simulink model "CACC"  (R2018a)
settings: Solver=VariableStepAuto  StartTime=0.0  StopTime=100  RelTol=1e-3
libraries: cstblocks x7
settings Model: Creator=uzeyi  LastModifiedBy=uzeyi

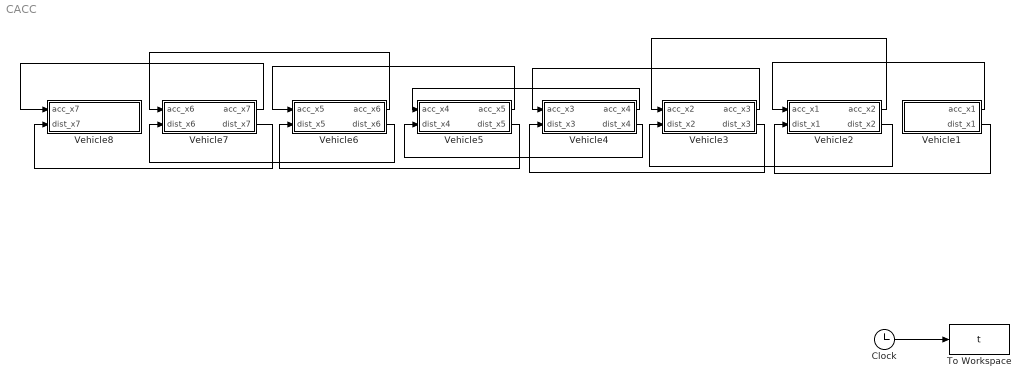
== system CACC ==
  Clock : Clock
  To Workspace : ToWorkspace  VariableName=t  SampleTime=-1
  Vehicle1 : Subsystem
  Vehicle2 : Subsystem
  Vehicle3 : Subsystem
  Vehicle4 : Subsystem
  Vehicle5 : Subsystem
  Vehicle6 : Subsystem
  Vehicle7 : Subsystem
  Vehicle8 : Subsystem
  wires:
  Vehicle1/2(dist_x1) -> Vehicle2/2(dist_x1)
  Clock/1 -> To Workspace/1
  Vehicle2/2(dist_x2) -> Vehicle3/2(dist_x2)
  Vehicle1/1("acc_x1 ") -> Vehicle2/1("acc_x1 ")
  Vehicle2/1(acc_x2) -> Vehicle3/1("acc_x2 ")
  Vehicle3/2(dist_x3) -> Vehicle4/2(dist_x3)
  Vehicle3/1(acc_x3) -> Vehicle4/1("acc_x3 ")
  Vehicle4/2(dist_x4) -> Vehicle5/2(dist_x4)
  Vehicle4/1(acc_x4) -> Vehicle5/1("acc_x4 ")
  Vehicle5/2(dist_x5) -> Vehicle6/2(dist_x5)
  Vehicle5/1(acc_x5) -> Vehicle6/1("acc_x5 ")
  Vehicle6/1(acc_x6) -> Vehicle7/1("acc_x6 ")
  Vehicle7/2(dist_x7) -> Vehicle8/2(dist_x7)
  Vehicle7/1(acc_x7) -> Vehicle8/1("acc_x7 ")
  Vehicle6/2(dist_x6) -> Vehicle7/2(dist_x6)

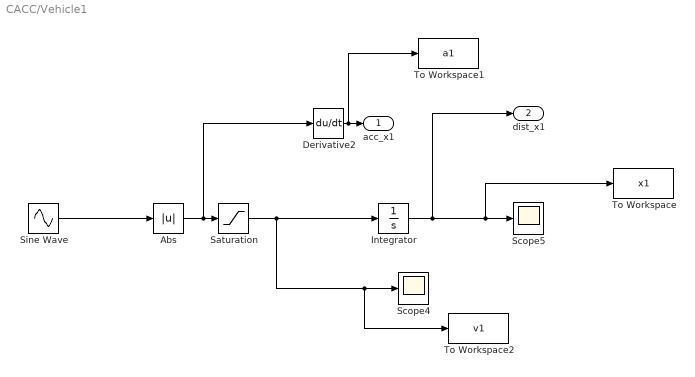
== system CACC/Vehicle1 ==
  Abs : Abs
  Derivative2 : Derivative
  Integrator : Integrator  InitialCondition=80
  Saturation : Saturate  UpperLimit=10  LowerLimit=5
  Scope4 : Scope
  Scope5 : Scope
  Sine Wave : Sin  Amplitude=10  SampleTime=0
  To Workspace : ToWorkspace  VariableName=x1  SampleTime=-1
  To Workspace1 : ToWorkspace  VariableName=a1  SampleTime=-1
  To Workspace2 : ToWorkspace  VariableName=v1  SampleTime=-1
  "acc_x1 " : Outport
  dist_x1 : Outport  Port=2
  wires:
  Sine Wave/1 -> Abs/1
  Saturation/1 -> To Workspace2/1, Scope4/1, Integrator/1
  Integrator/1 -> dist_x1/1, To Workspace/1, Scope5/1
  Derivative2/1 -> To Workspace1/1, "acc_x1 "/1
  Abs/1 -> Derivative2/1, Saturation/1

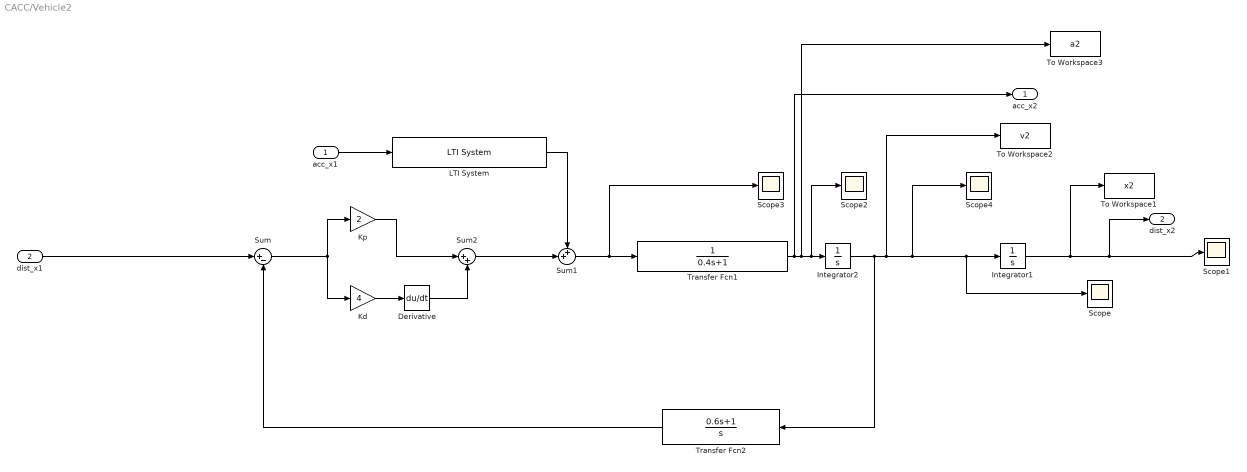
== system CACC/Vehicle2 ==
  "acc_x1 " : Inport
  dist_x1 : Inport  Port=2
  Derivative : Derivative
  Integrator1 : Integrator  InitialCondition=70  IgnoreLimit=on
  Integrator2 : Integrator  InitialCondition=1  IgnoreLimit=on
  Kd : Gain  Gain=4
  Kp : Gain  Gain=2
  LTI System : cstblocks/LTI System  sys=tf([0.4 1],[0.6 1],'InputDelay',0.3)  IC=[]
  Scope{,1..4} (5 alike) : Scope
  Sum : Sum  Inputs=|+-
  Sum1 : Sum  Inputs=++|
  Sum2 : Sum  Inputs=|++
  To Workspace1 : ToWorkspace  VariableName=x2  SampleTime=-1
  To Workspace2 : ToWorkspace  VariableName=v2  SampleTime=-1
  To Workspace3 : ToWorkspace  VariableName=a2  SampleTime=-1
  Transfer Fcn1 : TransferFcn  Denominator=[0.4 1 ]
  Transfer Fcn2 : TransferFcn  Numerator=[0.6 1]  Denominator=[1 0]
  acc_x2 : Outport
  dist_x2 : Outport  Port=2
  wires:
  Kd/1 -> Derivative/1
  LTI System/1 -> Sum1/1
  dist_x1/1 -> Sum/1
  Transfer Fcn1/1 -> acc_x2/1, To Workspace3/1, Scope2/1, Integrator2/1
  Transfer Fcn2/1 -> Sum/2
  Kp/1 -> Sum2/1
  "acc_x1 "/1 -> LTI System/1
  Integrator1/1 -> To Workspace1/1, dist_x2/1, Scope1/1
  Sum/1 -> Kp/1, Kd/1
  Integrator2/1 -> Transfer Fcn2/1, To Workspace2/1, Scope4/1, Scope/1, Integrator1/1
  Derivative/1 -> Sum2/2
  Sum1/1 -> Scope3/1, Transfer Fcn1/1
  Sum2/1 -> Sum1/2

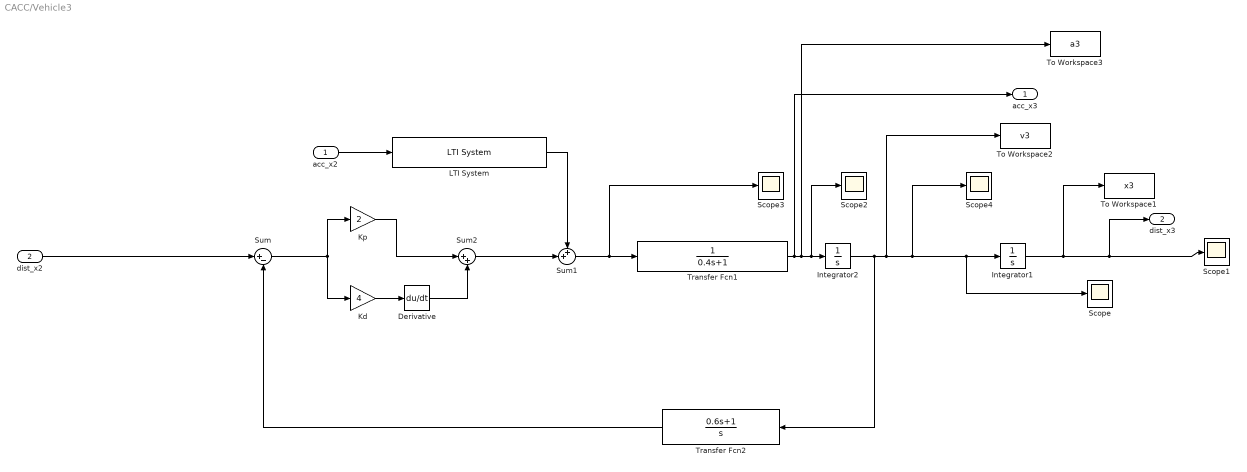
== system CACC/Vehicle3 ==
  "acc_x2 " : Inport
  dist_x2 : Inport  Port=2
  Derivative : Derivative
  Integrator1 : Integrator  InitialCondition=60  IgnoreLimit=on
  Integrator2 : Integrator  InitialCondition=1  IgnoreLimit=on
  Kd : Gain  Gain=4
  Kp : Gain  Gain=2
  LTI System : cstblocks/LTI System  sys=tf([0.4 1],[0.6 1],'InputDelay',0.3)  IC=[]
  Scope{,1..4} (5 alike) : Scope
  Sum : Sum  Inputs=|+-
  Sum1 : Sum  Inputs=++|
  Sum2 : Sum  Inputs=|++
  To Workspace1 : ToWorkspace  VariableName=x3  SampleTime=-1
  To Workspace2 : ToWorkspace  VariableName=v3  SampleTime=-1
  To Workspace3 : ToWorkspace  VariableName=a3  SampleTime=-1
  Transfer Fcn1 : TransferFcn  Denominator=[0.4 1 ]
  Transfer Fcn2 : TransferFcn  Numerator=[0.6 1]  Denominator=[1 0]
  acc_x3 : Outport
  dist_x3 : Outport  Port=2
  wires:
  Kd/1 -> Derivative/1
  LTI System/1 -> Sum1/1
  dist_x2/1 -> Sum/1
  Transfer Fcn1/1 -> acc_x3/1, To Workspace3/1, Scope2/1, Integrator2/1
  Transfer Fcn2/1 -> Sum/2
  Kp/1 -> Sum2/1
  "acc_x2 "/1 -> LTI System/1
  Integrator1/1 -> To Workspace1/1, dist_x3/1, Scope1/1
  Sum/1 -> Kp/1, Kd/1
  Integrator2/1 -> Transfer Fcn2/1, To Workspace2/1, Scope4/1, Scope/1, Integrator1/1
  Derivative/1 -> Sum2/2
  Sum1/1 -> Scope3/1, Transfer Fcn1/1
  Sum2/1 -> Sum1/2

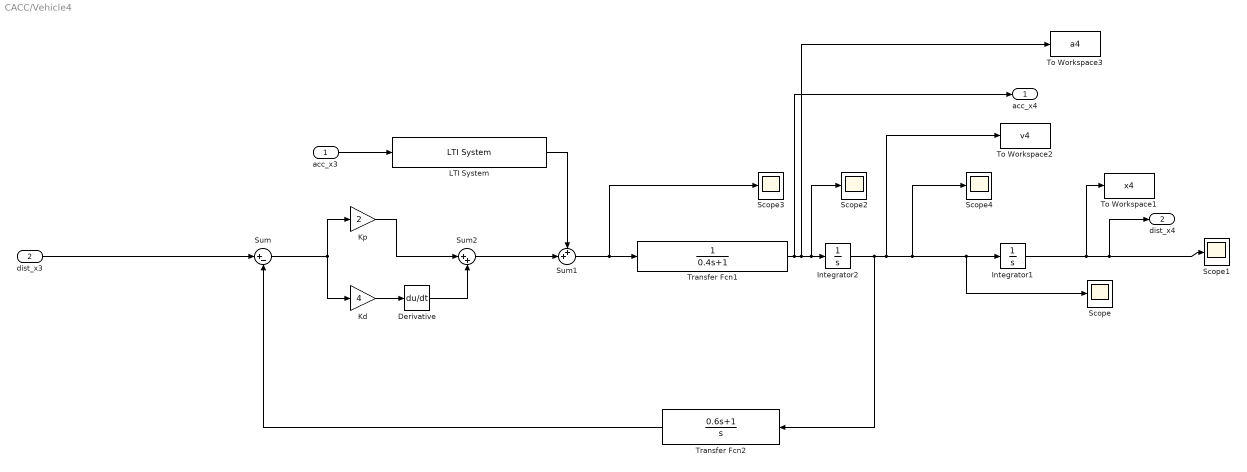
== system CACC/Vehicle4 ==
  "acc_x3 " : Inport
  dist_x3 : Inport  Port=2
  Derivative : Derivative
  Integrator1 : Integrator  InitialCondition=50  IgnoreLimit=on
  Integrator2 : Integrator  InitialCondition=1  IgnoreLimit=on
  Kd : Gain  Gain=4
  Kp : Gain  Gain=2
  LTI System : cstblocks/LTI System  sys=tf([0.4 1],[0.6 1],'InputDelay',0.3)  IC=[]
  Scope{,1..4} (5 alike) : Scope
  Sum : Sum  Inputs=|+-
  Sum1 : Sum  Inputs=++|
  Sum2 : Sum  Inputs=|++
  To Workspace1 : ToWorkspace  VariableName=x4  SampleTime=-1
  To Workspace2 : ToWorkspace  VariableName=v4  SampleTime=-1
  To Workspace3 : ToWorkspace  VariableName=a4  SampleTime=-1
  Transfer Fcn1 : TransferFcn  Denominator=[0.4 1 ]
  Transfer Fcn2 : TransferFcn  Numerator=[0.6 1]  Denominator=[1 0]
  acc_x4 : Outport
  dist_x4 : Outport  Port=2
  wires:
  Kd/1 -> Derivative/1
  LTI System/1 -> Sum1/1
  dist_x3/1 -> Sum/1
  Transfer Fcn1/1 -> acc_x4/1, To Workspace3/1, Scope2/1, Integrator2/1
  Transfer Fcn2/1 -> Sum/2
  Kp/1 -> Sum2/1
  "acc_x3 "/1 -> LTI System/1
  Integrator1/1 -> To Workspace1/1, dist_x4/1, Scope1/1
  Sum/1 -> Kp/1, Kd/1
  Integrator2/1 -> Transfer Fcn2/1, To Workspace2/1, Scope4/1, Scope/1, Integrator1/1
  Derivative/1 -> Sum2/2
  Sum1/1 -> Scope3/1, Transfer Fcn1/1
  Sum2/1 -> Sum1/2

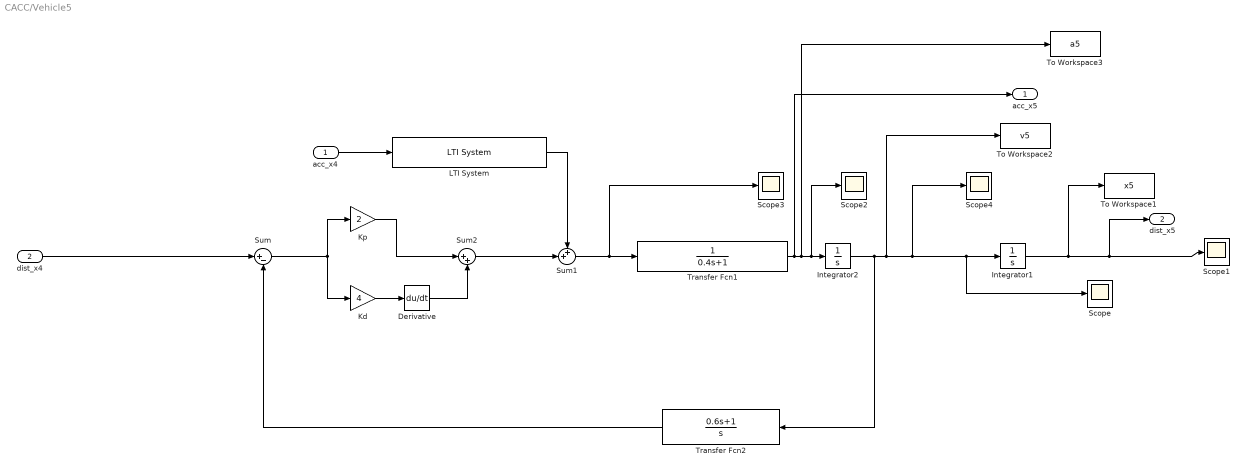
== system CACC/Vehicle5 ==
  "acc_x4 " : Inport
  dist_x4 : Inport  Port=2
  Derivative : Derivative
  Integrator1 : Integrator  InitialCondition=40  IgnoreLimit=on
  Integrator2 : Integrator  InitialCondition=1  IgnoreLimit=on
  Kd : Gain  Gain=4
  Kp : Gain  Gain=2
  LTI System : cstblocks/LTI System  sys=tf([0.4 1],[0.6 1],'InputDelay',0.3)  IC=[]
  Scope{,1..4} (5 alike) : Scope
  Sum : Sum  Inputs=|+-
  Sum1 : Sum  Inputs=++|
  Sum2 : Sum  Inputs=|++
  To Workspace1 : ToWorkspace  VariableName=x5  SampleTime=-1
  To Workspace2 : ToWorkspace  VariableName=v5  SampleTime=-1
  To Workspace3 : ToWorkspace  VariableName=a5  SampleTime=-1
  Transfer Fcn1 : TransferFcn  Denominator=[0.4 1 ]
  Transfer Fcn2 : TransferFcn  Numerator=[0.6 1]  Denominator=[1 0]
  acc_x5 : Outport
  dist_x5 : Outport  Port=2
  wires:
  Kd/1 -> Derivative/1
  LTI System/1 -> Sum1/1
  dist_x4/1 -> Sum/1
  Transfer Fcn1/1 -> acc_x5/1, To Workspace3/1, Scope2/1, Integrator2/1
  Transfer Fcn2/1 -> Sum/2
  Kp/1 -> Sum2/1
  "acc_x4 "/1 -> LTI System/1
  Integrator1/1 -> To Workspace1/1, dist_x5/1, Scope1/1
  Sum/1 -> Kp/1, Kd/1
  Integrator2/1 -> Transfer Fcn2/1, To Workspace2/1, Scope4/1, Scope/1, Integrator1/1
  Derivative/1 -> Sum2/2
  Sum1/1 -> Scope3/1, Transfer Fcn1/1
  Sum2/1 -> Sum1/2

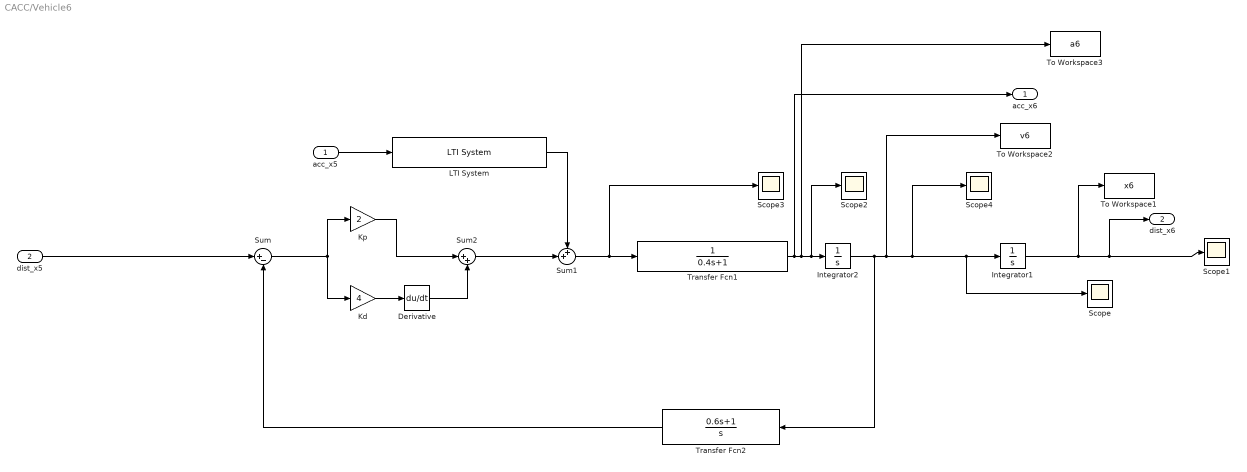
== system CACC/Vehicle6 ==
  "acc_x5 " : Inport
  dist_x5 : Inport  Port=2
  Derivative : Derivative
  Integrator1 : Integrator  InitialCondition=30  IgnoreLimit=on
  Integrator2 : Integrator  InitialCondition=1  IgnoreLimit=on
  Kd : Gain  Gain=4
  Kp : Gain  Gain=2
  LTI System : cstblocks/LTI System  sys=tf([0.4 1],[0.6 1],'InputDelay',0.3)  IC=[]
  Scope{,1..4} (5 alike) : Scope
  Sum : Sum  Inputs=|+-
  Sum1 : Sum  Inputs=++|
  Sum2 : Sum  Inputs=|++
  To Workspace1 : ToWorkspace  VariableName=x6  SampleTime=-1
  To Workspace2 : ToWorkspace  VariableName=v6  SampleTime=-1
  To Workspace3 : ToWorkspace  VariableName=a6  SampleTime=-1
  Transfer Fcn1 : TransferFcn  Denominator=[0.4 1 ]
  Transfer Fcn2 : TransferFcn  Numerator=[0.6 1]  Denominator=[1 0]
  acc_x6 : Outport
  dist_x6 : Outport  Port=2
  wires:
  Kd/1 -> Derivative/1
  LTI System/1 -> Sum1/1
  dist_x5/1 -> Sum/1
  Transfer Fcn1/1 -> acc_x6/1, To Workspace3/1, Scope2/1, Integrator2/1
  Transfer Fcn2/1 -> Sum/2
  Kp/1 -> Sum2/1
  "acc_x5 "/1 -> LTI System/1
  Integrator1/1 -> To Workspace1/1, dist_x6/1, Scope1/1
  Sum/1 -> Kp/1, Kd/1
  Integrator2/1 -> Transfer Fcn2/1, To Workspace2/1, Scope4/1, Scope/1, Integrator1/1
  Derivative/1 -> Sum2/2
  Sum1/1 -> Scope3/1, Transfer Fcn1/1
  Sum2/1 -> Sum1/2

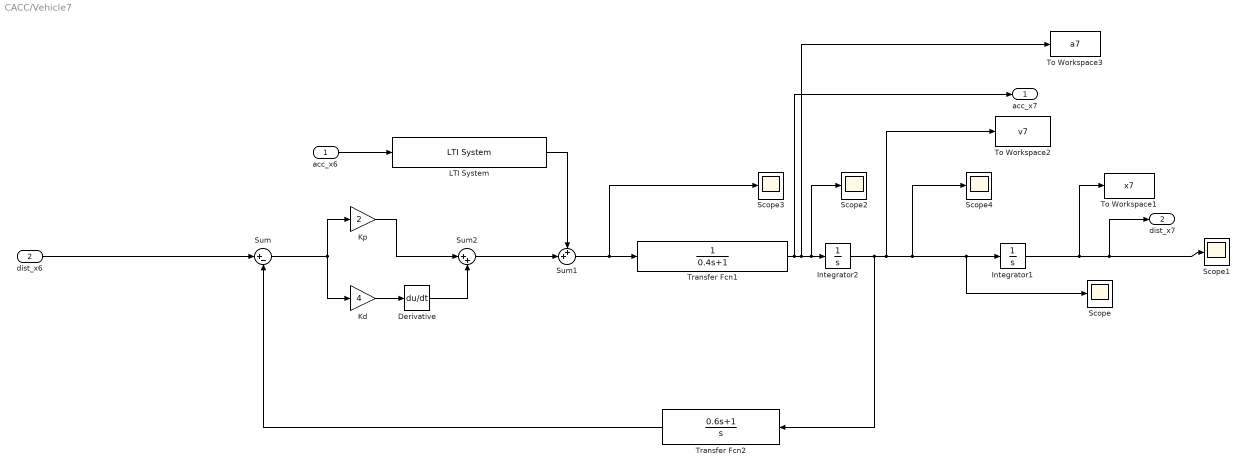
== system CACC/Vehicle7 ==
  "acc_x6 " : Inport
  dist_x6 : Inport  Port=2
  Derivative : Derivative
  Integrator1 : Integrator  InitialCondition=20  IgnoreLimit=on
  Integrator2 : Integrator  InitialCondition=1  IgnoreLimit=on
  Kd : Gain  Gain=4
  Kp : Gain  Gain=2
  LTI System : cstblocks/LTI System  sys=tf([0.4 1],[0.6 1],'InputDelay',0.3)  IC=[]
  Scope{,1..4} (5 alike) : Scope
  Sum : Sum  Inputs=|+-
  Sum1 : Sum  Inputs=++|
  Sum2 : Sum  Inputs=|++
  To Workspace1 : ToWorkspace  VariableName=x7  SampleTime=-1
  To Workspace2 : ToWorkspace  VariableName=v7  SampleTime=-1
  To Workspace3 : ToWorkspace  VariableName=a7  SampleTime=-1
  Transfer Fcn1 : TransferFcn  Denominator=[0.4 1 ]
  Transfer Fcn2 : TransferFcn  Numerator=[0.6 1]  Denominator=[1 0]
  acc_x7 : Outport
  dist_x7 : Outport  Port=2
  wires:
  Kd/1 -> Derivative/1
  LTI System/1 -> Sum1/1
  dist_x6/1 -> Sum/1
  Transfer Fcn1/1 -> acc_x7/1, To Workspace3/1, Scope2/1, Integrator2/1
  Transfer Fcn2/1 -> Sum/2
  Kp/1 -> Sum2/1
  "acc_x6 "/1 -> LTI System/1
  Integrator1/1 -> To Workspace1/1, dist_x7/1, Scope1/1
  Sum/1 -> Kp/1, Kd/1
  Integrator2/1 -> Transfer Fcn2/1, To Workspace2/1, Scope4/1, Scope/1, Integrator1/1
  Derivative/1 -> Sum2/2
  Sum1/1 -> Scope3/1, Transfer Fcn1/1
  Sum2/1 -> Sum1/2

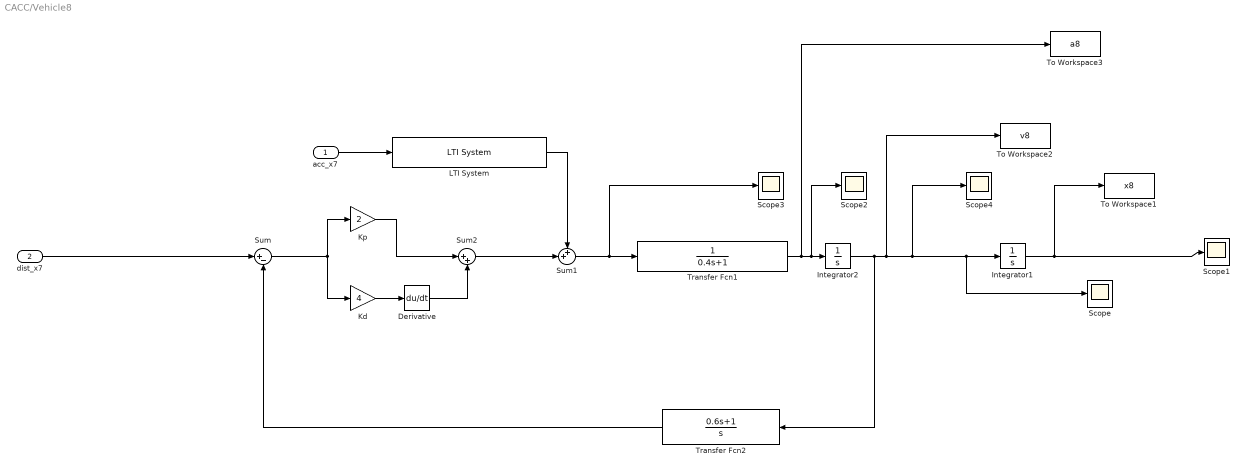
== system CACC/Vehicle8 ==
  "acc_x7 " : Inport
  dist_x7 : Inport  Port=2
  Derivative : Derivative
  Integrator1 : Integrator  InitialCondition=10  IgnoreLimit=on
  Integrator2 : Integrator  InitialCondition=1  IgnoreLimit=on
  Kd : Gain  Gain=4
  Kp : Gain  Gain=2
  LTI System : cstblocks/LTI System  sys=tf([0.4 1],[0.6 1],'InputDelay',0.3)  IC=[]
  Scope{,1..4} (5 alike) : Scope
  Sum : Sum  Inputs=|+-
  Sum1 : Sum  Inputs=++|
  Sum2 : Sum  Inputs=|++
  To Workspace1 : ToWorkspace  VariableName=x8  SampleTime=-1
  To Workspace2 : ToWorkspace  VariableName=v8  SampleTime=-1
  To Workspace3 : ToWorkspace  VariableName=a8  SampleTime=-1
  Transfer Fcn1 : TransferFcn  Denominator=[0.4 1 ]
  Transfer Fcn2 : TransferFcn  Numerator=[0.6 1]  Denominator=[1 0]
  wires:
  Kd/1 -> Derivative/1
  LTI System/1 -> Sum1/1
  dist_x7/1 -> Sum/1
  Transfer Fcn1/1 -> To Workspace3/1, Scope2/1, Integrator2/1
  Transfer Fcn2/1 -> Sum/2
  Kp/1 -> Sum2/1
  "acc_x7 "/1 -> LTI System/1
  Integrator1/1 -> To Workspace1/1, Scope1/1
  Sum/1 -> Kp/1, Kd/1
  Integrator2/1 -> Transfer Fcn2/1, To Workspace2/1, Scope4/1, Scope/1, Integrator1/1
  Derivative/1 -> Sum2/2
  Sum1/1 -> Scope3/1, Transfer Fcn1/1
  Sum2/1 -> Sum1/2
